simulink model "uav"  (R2016a)
settings: Solver=VariableStepAuto  StartTime=0.0  StopTime=700  RelTol=1e-3
values from neighbouring files (symbols this model uses):
  aim_point0 = [pp(1,10);pp(2,10)]    [test_ex_res.m]    (also in test_sim.m)
  p_out = [px_out';py_out']    [resamplepath.m]
  vAir = 10    [testpath.mat]
  vWind = [6.5 1]    [testpath.mat]
  x0 = pp(1,1)    [test_ex_res.m]    (also in test_sim.m)
  y0 = pp(2,1)    [test_ex_res.m]    (also in test_sim.m)
undefined symbols (not defined in the file or in its folder): h0
libraries: simulink x1
settings Model: Creator=aeagr  LastModifiedBy=aeagr

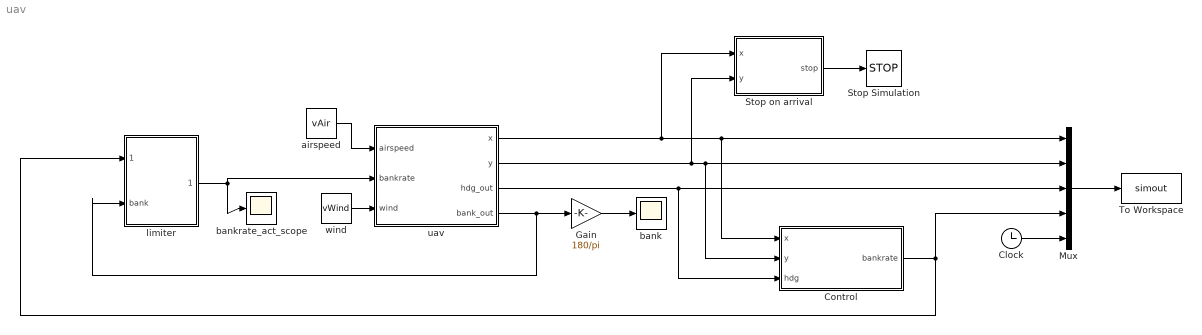
== system uav ==
  Clock : Clock
  Control : Subsystem  TreatAsAtomicUnit=on  SystemSampleTime=0.05
  Gain : Gain  Gain=180/pi
  Mux : Mux  Inputs=5
  Stop Simulation : Stop
  Stop on arrival : Subsystem
  To Workspace : ToWorkspace  VariableName=simout  SampleTime=-1
  airspeed : Constant  Value=vAir
  bank : Scope
  bankrate_act_scope : Scope
  limiter : Subsystem
  uav : Subsystem
  wind : Constant  Value=vWind
  wires:
  airspeed/1 -> uav/1(airspeed)
  wind/1 -> uav/3(wind)
  uav/1(x) -> Stop on arrival/1(x), Control/1(x), Mux/1
  uav/2(y) -> Stop on arrival/2(y), Control/2(y), Mux/2
  uav/3(hdg_out) -> Control/3(hdg), Mux/3
  Mux/1 -> To Workspace/1
  Clock/1 -> Mux/5
  uav/4(bank_out) -> limiter/2(bank), Gain/1
  limiter/1(bankrate_act) -> bankrate_act_scope/1, uav/2(bankrate)
  Gain/1 -> bank/1
  Control/1(bankrate) -> limiter/1(bankrate_req), Mux/4
  Stop on arrival/1(stop) -> Stop Simulation/1

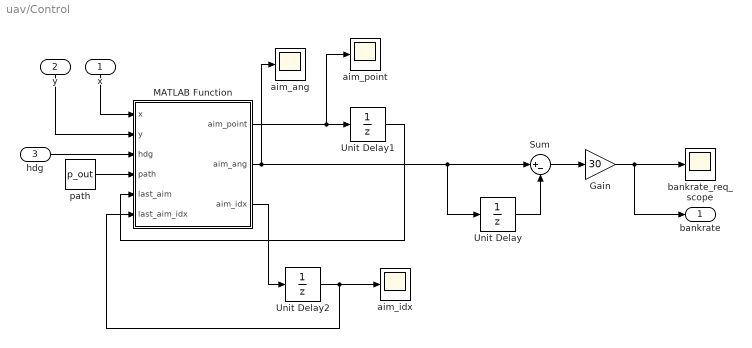
== system uav/Control ==
  x : Inport
  y : Inport  Port=2
  hdg : Inport  Port=3
  Gain : Gain  Gain=30
  MATLAB Function : MATLAB Function  TreatAsAtomicUnit=on
  Sum : Sum  Inputs=|+-
  Unit Delay : UnitDelay  SampleTime=-1
  Unit Delay1 : UnitDelay  InitialCondition=aim_point0  SampleTime=-1
  Unit Delay2 : UnitDelay  InitialCondition=1  SampleTime=-1
  aim_ang : Scope
  aim_idx : Scope
  aim_point : Scope
  bankrate_req_scope : Scope
  path : Constant  Value=p_out
  bankrate : Outport
  wires:
  hdg/1 -> MATLAB Function/3(hdg)
  path/1 -> MATLAB Function/4(path)
  MATLAB Function/2(aim_ang) -> Unit Delay/1, Sum/1, aim_ang/1
  Gain/1 -> bankrate/1, bankrate_req_scope/1
  x/1 -> MATLAB Function/1(x)
  MATLAB Function/1(aim_point) -> aim_point/1, Unit Delay1/1
  y/1 -> MATLAB Function/2(y)
  Sum/1 -> Gain/1
  Unit Delay/1 -> Sum/2
  Unit Delay1/1 -> MATLAB Function/5(last_aim)
  MATLAB Function/3(aim_idx) -> Unit Delay2/1
  Unit Delay2/1 -> aim_idx/1, MATLAB Function/6(last_aim_idx)

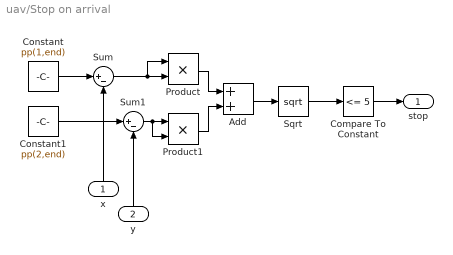
== system uav/Stop on arrival ==
  x : Inport
  y : Inport  Port=2
  Add : Sum
  Compare To Constant : simulink/Logic and Bit Operations/Compare To Constant  relop=<=  const=5  OutDataTypeStr=boolean
  Constant : Constant  Value=pp(1,end)
  Constant1 : Constant  Value=pp(2,end)
  Product : Product
  Product1 : Product
  Sqrt : Sqrt  SaturateOnIntegerOverflow=on
  Sum : Sum  Inputs=|+-
  Sum1 : Sum  Inputs=|+-
  stop : Outport
  wires:
  Product/1 -> Add/1
  Sqrt/1 -> Compare To Constant/1
  Constant/1 -> Sum/1
  Product1/1 -> Add/2
  Sum1/1 -> Product1/2, Product1/1
  y/1 -> Sum1/2
  x/1 -> Sum/2
  Compare To Constant/1 -> stop/1
  Add/1 -> Sqrt/1
  Constant1/1 -> Sum1/1
  Sum/1 -> Product/1, Product/2

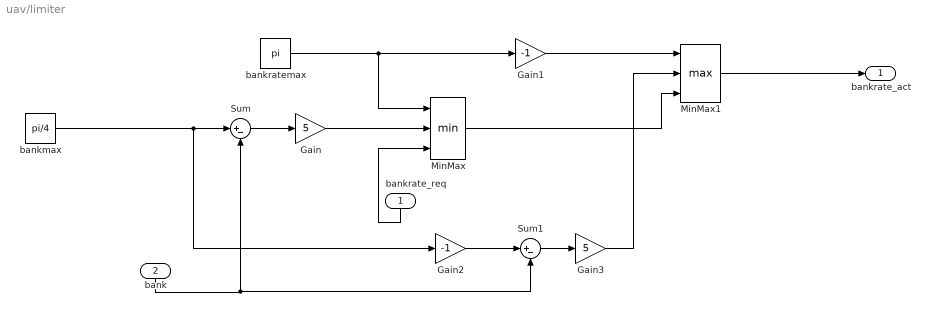
== system uav/limiter ==
  bankrate_req : Inport
  bank : Inport  Port=2
  Gain : Gain  Gain=5
  Gain1 : Gain  Gain=-1
  Gain2 : Gain  Gain=-1
  Gain3 : Gain  Gain=5
  MinMax : MinMax  Inputs=3
  MinMax1 : MinMax  Function=max  Inputs=3
  Sum : Sum  Inputs=|+-
  Sum1 : Sum  Inputs=|+-
  bankmax : Constant  Value=pi/4
  bankratemax : Constant  Value=pi
  bankrate_act : Outport
  wires:
  bankrate_req/1 -> MinMax/3
  bank/1 -> Sum1/2, Sum/2
  bankmax/1 -> Gain2/1, Sum/1
  Sum/1 -> Gain/1
  bankratemax/1 -> MinMax/1, Gain1/1
  Gain/1 -> MinMax/2
  MinMax/1 -> MinMax1/3
  Gain1/1 -> MinMax1/1
  MinMax1/1 -> bankrate_act/1
  Sum1/1 -> Gain3/1
  Gain2/1 -> Sum1/1
  Gain3/1 -> MinMax1/2

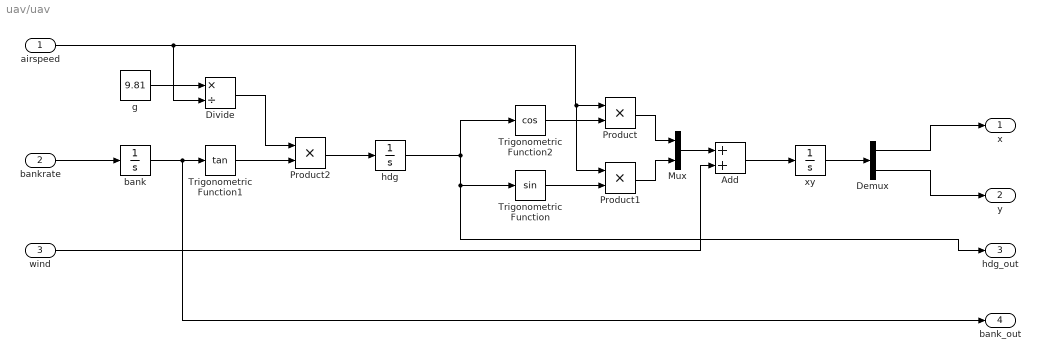
== system uav/uav ==
  airspeed : Inport
  bankrate : Inport  Port=2
  wind : Inport  Port=3
  Add : Sum
  Demux : Demux  Outputs=2
  Divide : Product  Inputs=*/
  Mux : Mux  Inputs=2
  Product : Product
  Product1 : Product
  Product2 : Product
  Trigonometric Function : Trigonometry
  Trigonometric Function1 : Trigonometry  Operator=tan
  Trigonometric Function2 : Trigonometry  Operator=cos
  bank : Integrator
  g : Constant  Value=9.81
  hdg : Integrator  InitialCondition=h0
  xy : Integrator  InitialCondition=[x0;y0]
  x : Outport
  y : Outport  Port=2
  hdg_out : Outport  Port=3
  bank_out : Outport  Port=4
  wires:
  hdg/1 -> hdg_out/1, Trigonometric Function/1, Trigonometric Function2/1
  bank/1 -> bank_out/1, Trigonometric Function1/1
  airspeed/1 -> Divide/2, Product1/1, Product/1
  Trigonometric Function2/1 -> Product/2
  Product2/1 -> hdg/1
  Trigonometric Function/1 -> Product1/2
  Demux/1 -> x/1
  Trigonometric Function1/1 -> Product2/2
  Add/1 -> xy/1
  Product/1 -> Mux/1
  Product1/1 -> Mux/2
  Mux/1 -> Add/1
  bankrate/1 -> bank/1
  xy/1 -> Demux/1
  wind/1 -> Add/2
  Demux/2 -> y/1
  g/1 -> Divide/1
  Divide/1 -> Product2/1

== matlab function uav/Control/MATLAB Function ==
  settings: sampleTime=0.1
  data: x input; aim_point output; y input; hdg input; path input; aim_ang output; last_aim input; last_aim_idx input; aim_idx output
function [aim_point,aim_ang,aim_idx] = follower(x,y,hdg,path,last_aim,last_aim_idx)
%#codegen

% predict ahead
d_pred = 3.0;
x_pred = x + d_pred*cos(hdg);
y_pred = y + d_pred*sin(hdg);

% limit path search for speed and robustness
path_rng = 5000;
start_idx = max(1,last_aim_idx-0.5*path_rng);
end_idx = min(size(path,2),last_aim_idx+path_rng);
local_path = path(1:2,start_idx:end_idx);

% choose closest point
path_dist = sum([local_path(1,:)-x_pred; local_path(2,:)-y_pred].^2);
[~,min_idx] = min(path_dist);
aim_point = local_path(:,min_idx);
aim_idx = start_idx+min_idx-1;

% filter
%aim_point = 0.99*aim_point + 0.01*last_aim;

aim_ang = atan2(aim_point(2)-y,aim_point(1)-x) - hdg;
if aim_ang>pi,
    aim_ang = aim_ang-2*pi;
elseif aim_ang<-pi,
    aim_ang = aim_ang+2*pi;
end
